simulink model "Pos_Vel_AccControl"  (Simulink 7.9)
settings: Solver=ode45  StartTime=0.0  StopTime=10.0  RelTol=1e-3
undefined symbols (not defined in the file): AccLimit, AccSourceSelect, DiscIntNeverNeededParam, KA, km, KP, kt, kTA, kTP, kTV, KV, LinePTs2Rpm, PosSourceSelect, Ra, TA, TauLimit, Ts, VelLimit, VelSourceSelect
libraries: powerlib_extras x4
settings Model: Creator=Administrator  LastModifiedBy=Administrator

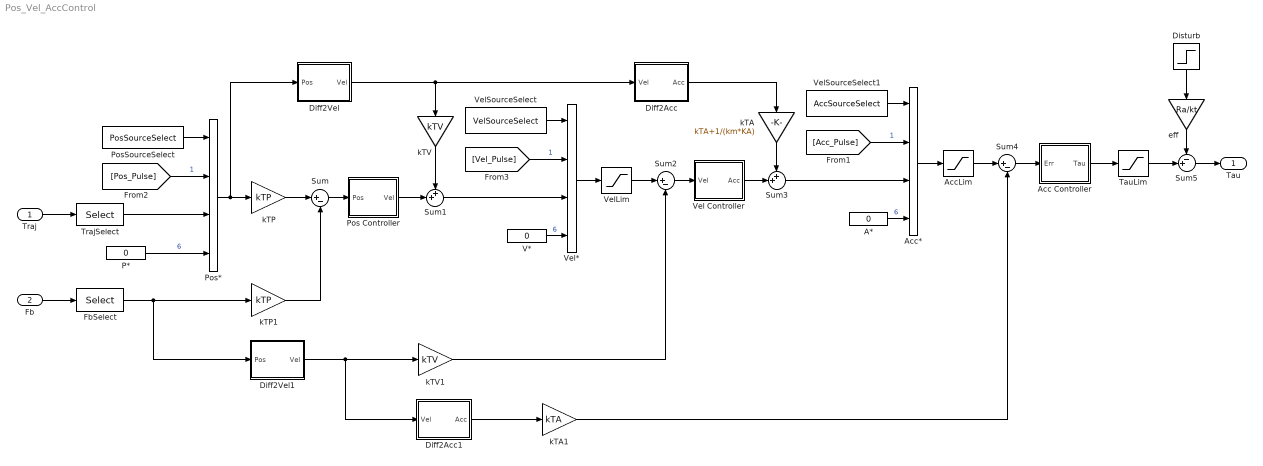
== system Pos_Vel_AccControl ==
  Traj : Inport
  Fb : Inport  Port=2
  A* : Constant  Value=0  SampleTime=Ts
  Acc Controller : Subsystem
  Acc* : MultiPortSwitch  zeroidx=off
  AccLim : Saturate  UpperLimit=AccLimit  LowerLimit=-AccLimit  SampleTime=Ts
  Diff2Acc : Subsystem
  Diff2Acc1 : Subsystem
  Diff2Vel : Subsystem
  Diff2Vel1 : Subsystem
  Disturb : Step  SampleTime=0
  FbSelect : Selector  InputPortWidth=6  IndexOptions=Index vector (dialog)  Indices=AxisNO  OutputSizes=1
  P* : Constant  Value=0  SampleTime=Ts
  Pos Controller : Subsystem
  Pos* : MultiPortSwitch  zeroidx=off  SampleTime=Ts
  PosSourceSelect : Constant  Value=PosSourceSelect  SampleTime=Ts
  Sum : Sum  Inputs=|+-  SampleTime=Ts
  Sum1 : Sum  Inputs=++|  SampleTime=Ts
  Sum2 : Sum  Inputs=|+-  SampleTime=Ts
  Sum3 : Sum  Inputs=++|  SampleTime=Ts
  Sum4 : Sum  Inputs=|+-  SampleTime=Ts
  Sum5 : Sum  Inputs=-+|  SampleTime=Ts
  TauLim : Saturate  UpperLimit=TauLimit  LowerLimit=-TauLimit  SampleTime=Ts
  TrajSelect : Selector  InputPortWidth=6  IndexOptions=Index vector (dialog)  Indices=AxisNO  OutputSizes=1
  V* : Constant  Value=0  SampleTime=Ts
  Vel Controller : Subsystem
  Vel* : MultiPortSwitch  zeroidx=off
  VelLim : Saturate  UpperLimit=VelLimit  LowerLimit=-VelLimit  SampleTime=Ts
  VelSourceSelect : Constant  Value=VelSourceSelect  SampleTime=Ts
  VelSourceSelect1 : Constant  Value=AccSourceSelect  SampleTime=Ts
  eff : Gain  Gain=Ra/kt  SampleTime=Ts
  kTA : Gain  Gain=kTA+1/(km*KA)  SampleTime=Ts
  kTA1 : Gain  Gain=kTA  SampleTime=Ts
  kTP : Gain  Gain=kTP  SampleTime=Ts
  kTP1 : Gain  Gain=kTP  SampleTime=Ts
  kTV : Gain  Gain=kTV  SampleTime=Ts
  kTV1 : Gain  Gain=kTV  SampleTime=Ts
  Tau : Outport
  wires:
  [Pos_Pulse] -> Pos*/2  "1"
  TrajSelect/1 -> Pos*/3
  P*/1 -> Pos*/4  "6"
  PosSourceSelect/1 -> Pos*/1
  Traj/1 -> TrajSelect/1
  Pos*/1 -> kTP/1, Diff2Vel/1(Pos)
  kTP/1 -> Sum/1
  Sum/1 -> Pos Controller/1(Pos)
  Pos Controller/1(Vel) -> Sum1/2
  kTV/1 -> Sum1/1
  Diff2Vel/1(Vel) -> kTV/1, Diff2Acc/1(Vel)
  VelLim/1 -> Sum2/1
  Vel Controller/1(Acc) -> Sum3/2
  Diff2Acc/1(Acc) -> kTA/1
  kTA/1 -> Sum3/1
  V*/1 -> Vel*/4  "6"
  [Vel_Pulse] -> Vel*/2  "1"
  Vel*/1 -> VelLim/1
  VelSourceSelect/1 -> Vel*/1
  Sum1/1 -> Vel*/3
  AccLim/1 -> Sum4/1
  Sum4/1 -> Acc Controller/1(Err)
  Sum2/1 -> Vel Controller/1(Vel)
  Acc Controller/1(Tau) -> TauLim/1
  Sum5/1 -> Tau/1
  Fb/1 -> FbSelect/1
  FbSelect/1 -> kTP1/1, Diff2Vel1/1(Pos)
  kTP1/1 -> Sum/2
  Diff2Vel1/1(Vel) -> kTV1/1, Diff2Acc1/1(Vel)
  kTV1/1 -> Sum2/2
  Diff2Acc1/1(Acc) -> kTA1/1
  kTA1/1 -> Sum4/2
  A*/1 -> Acc*/4  "6"
  [Acc_Pulse] -> Acc*/2  "1"
  VelSourceSelect1/1 -> Acc*/1
  Sum3/1 -> Acc*/3
  Acc*/1 -> AccLim/1
  eff/1 -> Sum5/1
  Disturb/1 -> eff/1
  TauLim/1 -> Sum5/2

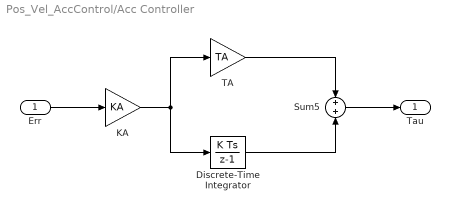
== system Pos_Vel_AccControl/Acc Controller ==
  Err : Inport
  Discrete-Time Integrator : DiscreteIntegrator  SampleTime=Ts  ICPrevOutput=DiscIntNeverNeededParam  ICPrevScaledInput=DiscIntNeverNeededParam
  KA : Gain  Gain=KA  SampleTime=Ts
  Sum5 : Sum  Inputs=+|+
  TA : Gain  Gain=TA  SampleTime=Ts
  Tau : Outport
  wires:
  TA/1 -> Sum5/1
  Discrete-Time Integrator/1 -> Sum5/2
  KA/1 -> TA/1, Discrete-Time Integrator/1
  Err/1 -> KA/1
  Sum5/1 -> Tau/1

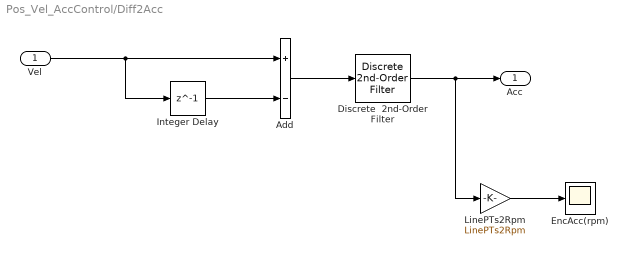
== system Pos_Vel_AccControl/Diff2Acc ==
  Vel : Inport
  Add : Sum  Inputs=+-
  Discrete  2nd-Order Filter : powerlib_extras/Discrete  Control Blocks/Discrete  2nd-Order Filter  FilterType=Lowpass  Fo=200  Zeta=0.707  Ts=Ts  Initialize=off  Vac_Init=[0.8 -25 60]  Vdc_Init=-0.4  PlotResponse=off  param1=[1 5000 10]
  EncAcc(rpm) : Scope
      settings: SaveName=ScopeData33
  Integer Delay : Delay  DelayLength=1  InputProcessing=Inherited
  LinePTs2Rpm : Gain  Gain=LinePTs2Rpm
  Acc : Outport
  wires:
  Add/1 -> Discrete  2nd-Order Filter/1
  Discrete  2nd-Order Filter/1 -> Acc/1, LinePTs2Rpm/1
  Vel/1 -> Integer Delay/1, Add/1
  Integer Delay/1 -> Add/2
  LinePTs2Rpm/1 -> EncAcc(rpm)/1

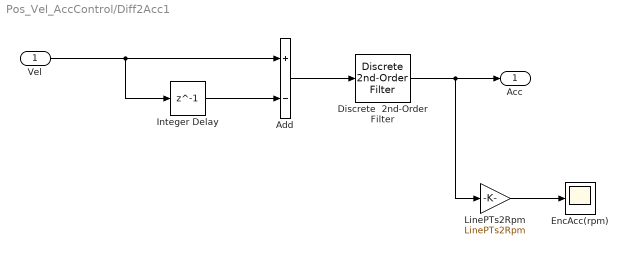
== system Pos_Vel_AccControl/Diff2Acc1 ==
  Vel : Inport
  Add : Sum  Inputs=+-
  Discrete  2nd-Order Filter : powerlib_extras/Discrete  Control Blocks/Discrete  2nd-Order Filter  FilterType=Lowpass  Fo=200  Zeta=0.707  Ts=Ts  Initialize=off  Vac_Init=[0.8 -25 60]  Vdc_Init=-0.4  PlotResponse=off  param1=[1 5000 10]
  EncAcc(rpm) : Scope
      settings: SaveName=ScopeData33
  Integer Delay : Delay  DelayLength=1  InputProcessing=Inherited
  LinePTs2Rpm : Gain  Gain=LinePTs2Rpm
  Acc : Outport
  wires:
  Add/1 -> Discrete  2nd-Order Filter/1
  Discrete  2nd-Order Filter/1 -> Acc/1, LinePTs2Rpm/1
  Vel/1 -> Integer Delay/1, Add/1
  Integer Delay/1 -> Add/2
  LinePTs2Rpm/1 -> EncAcc(rpm)/1

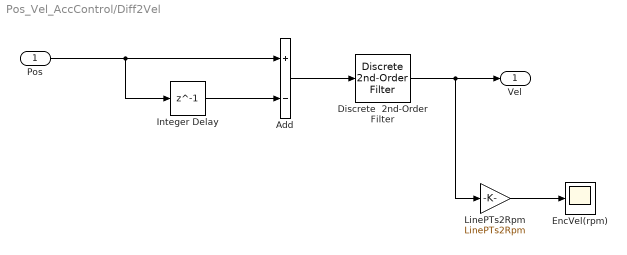
== system Pos_Vel_AccControl/Diff2Vel ==
  Pos : Inport
  Add : Sum  Inputs=+-
  Discrete  2nd-Order Filter : powerlib_extras/Discrete  Control Blocks/Discrete  2nd-Order Filter  FilterType=Lowpass  Fo=200  Zeta=0.707  Ts=Ts  Initialize=off  Vac_Init=[0.8 -25 60]  Vdc_Init=-0.4  PlotResponse=off  param1=[1 5000 10]
  EncVel(rpm) : Scope
      settings: SaveName=ScopeData33
  Integer Delay : Delay  DelayLength=1  InputProcessing=Inherited
  LinePTs2Rpm : Gain  Gain=LinePTs2Rpm
  Vel : Outport
  wires:
  Add/1 -> Discrete  2nd-Order Filter/1
  Discrete  2nd-Order Filter/1 -> Vel/1, LinePTs2Rpm/1
  Pos/1 -> Integer Delay/1, Add/1
  Integer Delay/1 -> Add/2
  LinePTs2Rpm/1 -> EncVel(rpm)/1

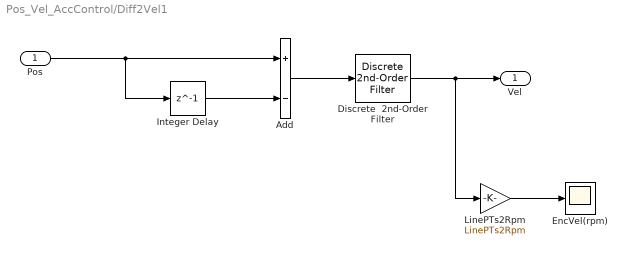
== system Pos_Vel_AccControl/Diff2Vel1 ==
  Pos : Inport
  Add : Sum  Inputs=+-
  Discrete  2nd-Order Filter : powerlib_extras/Discrete  Control Blocks/Discrete  2nd-Order Filter  FilterType=Lowpass  Fo=200  Zeta=0.707  Ts=Ts  Initialize=off  Vac_Init=[0.8 -25 60]  Vdc_Init=-0.4  PlotResponse=off  param1=[1 5000 10]
  EncVel(rpm) : Scope
      settings: SaveName=ScopeData33
  Integer Delay : Delay  DelayLength=1  InputProcessing=Inherited
  LinePTs2Rpm : Gain  Gain=LinePTs2Rpm
  Vel : Outport
  wires:
  Add/1 -> Discrete  2nd-Order Filter/1
  Discrete  2nd-Order Filter/1 -> Vel/1, LinePTs2Rpm/1
  Pos/1 -> Integer Delay/1, Add/1
  Integer Delay/1 -> Add/2
  LinePTs2Rpm/1 -> EncVel(rpm)/1

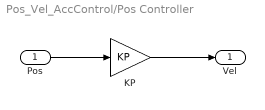
== system Pos_Vel_AccControl/Pos Controller ==
  Pos : Inport
  KP : Gain  Gain=KP  SampleTime=Ts
  Vel : Outport
  wires:
  Pos/1 -> KP/1
  KP/1 -> Vel/1

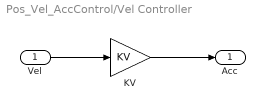
== system Pos_Vel_AccControl/Vel Controller ==
  Vel : Inport
  KV : Gain  Gain=KV  SampleTime=Ts
  Acc : Outport
  wires:
  Vel/1 -> KV/1
  KV/1 -> Acc/1
